simulink model "M3modellSOMFUNKAR2019"  (Simulink 10.0)
settings: Solver=FixedStepDiscrete  StartTime=0.0  StopTime=20  FixedStep=h  RelTol=1e-3  EnableMultiTasking=on
values from neighbouring files (symbols this model uses):
  Ad = expm(A*Ts)    [M3.m]
  Bd = Bd_int    [M3.m]
  C = [0 1 0 0 1]    [M3.m]
  h = 0.001    [M3.m]
  K_fb = Klqr(:,1:length(Ad))    [M3.m]
  K_I = Klqr(:,6)    [M3.m]
  R1 = sigma_val_v    [M3.m]
  sigma_val_noise1 = double(solve(Phi_T==PoR/100,sigma))    [M3.m]
  sigma_val_noise2 = double(solve(Phi_T==PoR/100,sigma))    [M3.m]
  sigma_val_T = double(solve(Phi_T==PoR/100,sigma))    [M3.m]
  sigma_val_v = double(solve(Phi_v==PoR/100,sigma))    [M3.m]
undefined symbols (not defined in the file or in its folder): DiscIntNeverNeededParam, L_CT
settings Model: LogicAnalyzerSignalOrdering=c674b985-68a9-48ad-8755-6330c9de9e3f,132b132a-59eb-4269-9237-96aa76f05394,aa8030fc-a0bd-4224-a17d-a78a186524c0,55d7cc7c-c459-483a-bb1c-a337b4a327d9,e7d90428-d509-4e49-a321-668cc670d116,777044fe-aef5-48a1-aa55-6c52ec9cb220  Creator=tw  LastModifiedBy=albin
settings DataIOCC: LimitDataPoints=on  MaxDataPoints=1000000
settings OptimizationCC: ExpressionDepthLimit=2147483647  InitFltsAndDblsToZero=on
settings DebuggingCC: SaveWithParameterizedLinksMsg=none  SolverPrmCheckMsg=warning  FcnCallInpInsideContextMsg=warning  StateNameClashWarn=warning
settings GRTTargetCC: TargetFcnLib=ansi_tfl_tmw.mat
settings ConfigComp: CovExternalEMLEnable=off

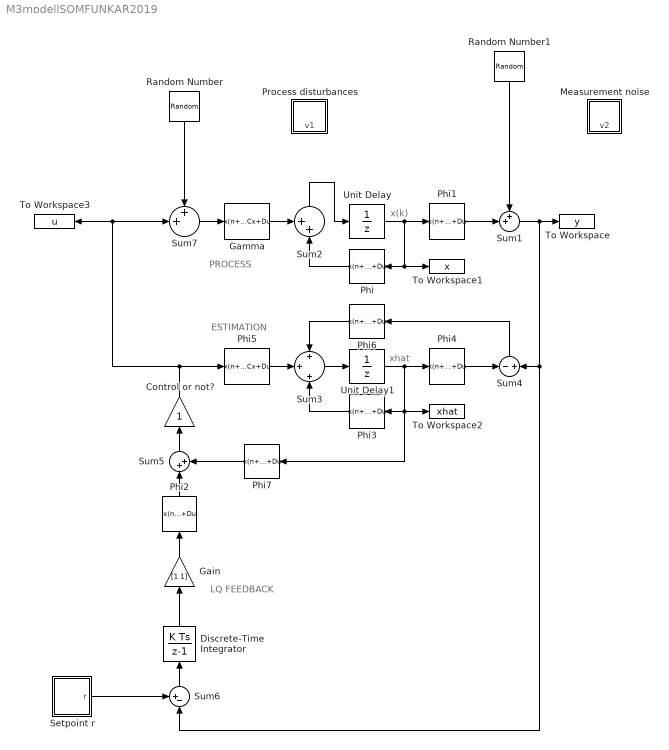
== system M3modellSOMFUNKAR2019 ==
  note: x(k)
  note: xhat
  note: PROCESS
  note: LQ FEEDBACK
  note: ESTIMATION
  Control or not? : Gain
  Discrete-Time Integrator : DiscreteIntegrator  SampleTime=-1  ICPrevOutput=DiscIntNeverNeededParam  ICPrevScaledInput=DiscIntNeverNeededParam
  Gain : Gain  Gain=[1 1]
  Gamma : DiscreteStateSpace  A=[]  B=[]  C=[]  D=Bd  SampleTime=-1  mask(Vector gain){}
      mask Display: disp('Bd')
  Measurement noise : Subsystem
  Phi : DiscreteStateSpace  A=[]  B=[]  C=[]  D=Ad  SampleTime=-1  mask(Vector gain){}
      mask Display: disp('Ad')
  Phi1 : DiscreteStateSpace  A=[]  B=[]  C=[]  D=C  SampleTime=-1  mask(Vector gain){}
      mask Display: disp('C')
  Phi2 : DiscreteStateSpace  A=[]  B=[]  C=[]  D=-K_I  SampleTime=-1  mask(Vector gain){}
      mask Display: disp('-K_I')
  Phi3 : DiscreteStateSpace  A=[]  B=[]  C=[]  D=Ad  SampleTime=-1  mask(Vector gain){}
      mask Display: disp('Ad')
  Phi4 : DiscreteStateSpace  A=[]  B=[]  C=[]  D=C  SampleTime=-1  mask(Vector gain){}
      mask Display: disp('C')
  Phi5 : DiscreteStateSpace  A=[]  B=[]  C=[]  D=Bd  SampleTime=-1  mask(Vector gain){}
      mask Display: disp('Bd')
  Phi6 : DiscreteStateSpace  A=[]  B=[]  C=[]  D=L_CT  SampleTime=-1  mask(Vector gain){}
      mask Display: disp('L')
  Phi7 : DiscreteStateSpace  A=[]  B=[]  C=[]  D=-K_fb  SampleTime=-1  mask(Vector gain){}
      mask Display: disp('-K_fb')
  Process disturbances : Subsystem
  Random Number : RandomNumber  Variance=[sigma_val_v sigma_val_T]  SampleTime=h
  Random Number1 : RandomNumber  Variance=[sigma_val_noise1 sigma_val_noise2]  SampleTime=h
  Setpoint r : Subsystem
  Sum1 : Sum  Inputs=++|
  Sum2 : Sum  Inputs=++|
  Sum3 : Sum  Inputs=+|+|+
  Sum4 : Sum  Inputs=-|+
  Sum5 : Sum  Inputs=|++
  Sum6 : Sum  Inputs=+-|
  Sum7 : Sum  Inputs=++|
  To Workspace : ToWorkspace  VariableName=y  SampleTime=-1
  To Workspace1 : ToWorkspace  VariableName=x  SampleTime=-1
  To Workspace2 : ToWorkspace  VariableName=xhat  SampleTime=-1
  To Workspace3 : ToWorkspace  VariableName=u  SampleTime=-1
  Unit Delay : UnitDelay  SampleTime=-1  HasFrameUpgradeWarning=on
  Unit Delay1 : UnitDelay  SampleTime=-1  HasFrameUpgradeWarning=on
  wires:
  Sum2/1 -> Unit Delay/1
  Unit Delay/1 -> Phi1/1, Phi/1, To Workspace1/1
  Phi1/1 -> Sum1/2
  Sum1/1 -> Sum6/2, Sum4/2, To Workspace/1
  Phi/1 -> Sum2/2
  Sum3/1 -> Unit Delay1/1
  Unit Delay1/1 -> Phi4/1, Phi7/1, Phi3/1, To Workspace2/1
  Phi5/1 -> Sum3/2
  Phi3/1 -> Sum3/3
  Phi4/1 -> Sum4/1
  Sum4/1 -> Phi6/1
  Phi6/1 -> Sum3/1
  Control or not?/1 -> Phi5/1, Sum7/2, To Workspace3/1
  Discrete-Time Integrator/1 -> Gain/1
  Setpoint r/1(r) -> Sum6/1
  Sum6/1 -> Discrete-Time Integrator/1
  Sum5/1 -> Control or not?/1
  Phi2/1 -> Sum5/1
  Phi7/1 -> Sum5/2
  Gamma/1 -> Sum2/1
  Sum7/1 -> Gamma/1
  Random Number/1 -> Sum7/1
  Random Number1/1 -> Sum1/1
  Gain/1 -> Phi2/1

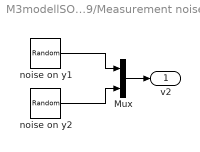
== system M3modellSOMFUNKAR2019/Measurement noise ==
  Mux : Mux  Inputs=2
  noise on y1 : RandomNumber  Variance=sigma_val_noise1  Seed=5  SampleTime=h
  noise on y2 : RandomNumber  Variance=sigma_val_noise2  Seed=4  SampleTime=h
  v2 : Outport
  wires:
  noise on y1/1 -> Mux/1
  noise on y2/1 -> Mux/2
  Mux/1 -> v2/1

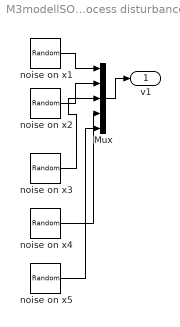
== system M3modellSOMFUNKAR2019/Process disturbances ==
  Mux : Mux  Inputs=5
  noise on x1 : RandomNumber  Variance=R1(1,1)  Seed=3  SampleTime=h
  noise on x{2..5} (4 alike) : RandomNumber  Variance=R1  Seed=2  SampleTime=h
  v1 : Outport
  wires:
  noise on x1/1 -> Mux/1
  noise on x2/1 -> Mux/2
  Mux/1 -> v1/1
  noise on x3/1 -> Mux/3
  noise on x4/1 -> Mux/4
  noise on x5/1 -> Mux/5

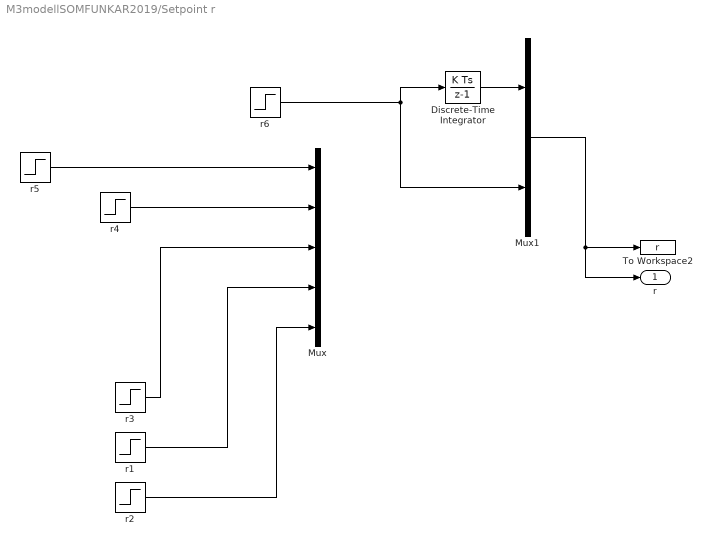
== system M3modellSOMFUNKAR2019/Setpoint r ==
  Discrete-Time Integrator : DiscreteIntegrator  SampleTime=-1  ICPrevOutput=DiscIntNeverNeededParam  ICPrevScaledInput=DiscIntNeverNeededParam
  Mux : Mux  Inputs=5
  Mux1 : Mux  Inputs=2
  To Workspace2 : ToWorkspace  VariableName=r  SampleTime=-1
  r{1,3..5} (4 alike) : Step  Time=0  After=0  SampleTime=h
  r2 : Step  Time=5  Before=10  After=100  SampleTime=h
  r6 : Step  Time=0.5  Before=10  After=100  SampleTime=h
  r : Outport
  wires:
  r1/1 -> Mux/4
  r2/1 -> Mux/5
  r3/1 -> Mux/3
  r4/1 -> Mux/2
  r5/1 -> Mux/1
  r6/1 -> Mux1/2, Discrete-Time Integrator/1
  Mux1/1 -> r/1, To Workspace2/1
  Discrete-Time Integrator/1 -> Mux1/1
